simulink model "model2"  (R2020a)
settings: Solver=VariableStepAuto  StartTime=0.0  StopTime=100  RelTol=1e-3
settings Model: Creator=11196  LastModifiedBy=11196

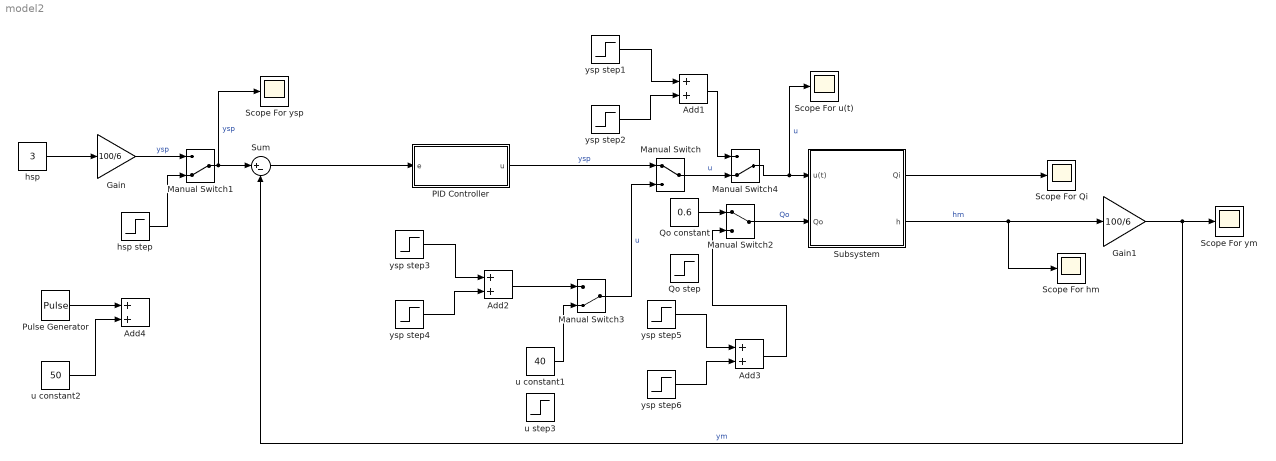
== system model2 ==
  Add{1..4} (4 alike) : Sum
  Gain : Gain  Gain=100/6
  Gain1 : Gain  Gain=100/6
  Manual Switch : ManualSwitch
  Manual Switch1 : ManualSwitch  CurrentSetting=0
  Manual Switch2 : ManualSwitch
  Manual Switch3 : ManualSwitch  CurrentSetting=0
  Manual Switch4 : ManualSwitch  CurrentSetting=0
  PID Controller : Subsystem
  Pulse Generator : DiscretePulseGenerator  PulseType=Time based  Amplitude=10  Period=20  PulseWidth=50
  Qo constant : Constant  Value=0.6
  Qo step : Step  Time=20  Before=0.6  After=0.72  SampleTime=0
  Scope For Qi : Scope
  Scope For hm : Scope
  Scope For u(t) : Scope
  Scope For ym : Scope
  Scope For ysp : Scope
  Subsystem : Subsystem
  Sum : Sum  Inputs=|+-
  hsp : Constant  Value=3
  hsp step : Step  Time=20  Before=50  After=59  SampleTime=0
  u constant1 : Constant  Value=40
  u constant2 : Constant  Value=50
  u step3 : Step  Time=20  Before=40  After=48  SampleTime=0
  ysp step1 : Step  Time=20  Before=50  After=60  SampleTime=0
  ysp step2 : Step  Time=30  Before=60  After=50  SampleTime=0
  ysp step3 : Step  Time=20  Before=40  After=48  SampleTime=0
  ysp step4 : Step  Time=22  After=-8  SampleTime=0
  ysp step5 : Step  Time=20  Before=0.6  After=0.72  SampleTime=0
  ysp step6 : Step  Time=22  After=-0.12  SampleTime=0
  wires:
  Manual Switch1/1 -> Scope For ysp/1, Sum/1  "ysp"
  Qo constant/1 -> Manual Switch2/1
  Subsystem/1(Qi) -> Scope For Qi/1
  Gain/1 -> Manual Switch1/1  "ysp"
  hsp/1 -> Gain/1
  Gain1/1 -> Sum/2, Scope For ym/1  "ym"
  Subsystem/2(h) -> Scope For hm/1, Gain1/1  "hm"
  Manual Switch2/1 -> Subsystem/2(Qo)  "Qo"
  Manual Switch3/1 -> Manual Switch/2  "u"
  Manual Switch/1 -> Manual Switch4/2  "u"
  Manual Switch4/1 -> Scope For u(t)/1, Subsystem/1(u(t))  "u"
  ysp step1/1 -> Add1/1
  ysp step2/1 -> Add1/2
  Add1/1 -> Manual Switch4/1
  ysp step4/1 -> Add2/2
  ysp step3/1 -> Add2/1
  Add2/1 -> Manual Switch3/1
  u constant1/1 -> Manual Switch3/2
  ysp step5/1 -> Add3/1
  ysp step6/1 -> Add3/2
  Add3/1 -> Manual Switch2/2
  PID Controller/1(u) -> Manual Switch/1  "ysp"
  Sum/1 -> PID Controller/1(e)
  Pulse Generator/1 -> Add4/1
  u constant2/1 -> Add4/2
  hsp step/1 -> Manual Switch1/2

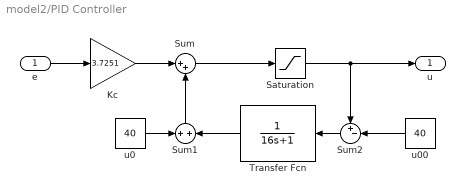
== system model2/PID Controller ==
  e : Inport
  Kc : Gain  Gain=3.7251
  Saturation : Saturate  UpperLimit=100  LowerLimit=0
  Sum : Sum  Inputs=|++
  Sum1 : Sum  Inputs=+|+
  Sum2 : Sum  Inputs=+-|
  Transfer Fcn : TransferFcn  Denominator=[16 1]
  u0 : Constant  Value=40
  u00 : Constant  Value=40
  u : Outport
  wires:
  e/1 -> Kc/1
  Kc/1 -> Sum/1
  Sum/1 -> Saturation/1
  Saturation/1 -> Sum2/1, u/1
  u00/1 -> Sum2/2
  u0/1 -> Sum1/1
  Sum2/1 -> Transfer Fcn/1
  Transfer Fcn/1 -> Sum1/2
  Sum1/1 -> Sum/2

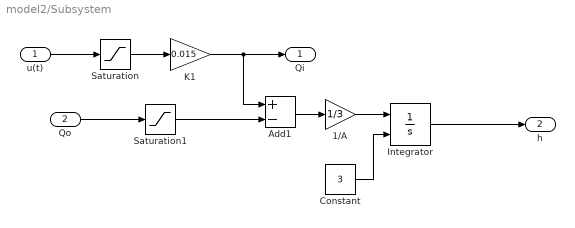
== system model2/Subsystem ==
  u(t) : Inport
  Qo : Inport  Port=2
  1/A : Gain  Gain=1/3
  Add1 : Sum  Inputs=+-
  Constant : Constant  Value=3
  Integrator : Integrator  InitialConditionSource=external  InitialCondition=3  LimitOutput=on  UpperSaturationLimit=6  LowerSaturationLimit=0
  K1 : Gain  Gain=0.015
  Saturation : Saturate  UpperLimit=100  LowerLimit=0
  Saturation1 : Saturate  UpperLimit=1  LowerLimit=0
  Qi : Outport
  h : Outport  Port=2
  wires:
  Saturation/1 -> K1/1
  Add1/1 -> 1/A/1
  1/A/1 -> Integrator/1
  Constant/1 -> Integrator/2
  u(t)/1 -> Saturation/1
  Integrator/1 -> h/1
  K1/1 -> Add1/1, Qi/1
  Qo/1 -> Saturation1/1
  Saturation1/1 -> Add1/2
